simulink model "exemple_thermo_1"  (Simulink 8.1)
settings: Solver=ode4  StartTime=0.0  StopTime=10.0  FixedStep=1e-4  RelTol=1e-3
values from neighbouring files (symbols this model uses):
  Cp = 1000    [init_modele_thermo.m]
  Cv = 713    [init_modele_thermo.m]
  P0 = 1e5    (= 100000)    [init_modele_thermo.m]
  P1 = 1.05e5    (= 105000)    [init_modele_thermo.m]
  Pinit = 1e5    (= 100000)    [init_modele_thermo.m]
  r = 286.68    [init_modele_thermo.m]
  S_amont = pi/4*(5e-3)^2    (= 1.96349540849e-05)    [init_modele_thermo.m]
  S_aval = pi/4*(5e-3)^2    (= 1.96349540849e-05)    [init_modele_thermo.m]
  T0 = 300    [init_modele_thermo.m]
  T1 = 373    [init_modele_thermo.m]
  Tinit = 300    [init_modele_thermo.m]
  V = 1e-3    (= 0.001)    [init_modele_thermo.m]
settings Model: Creator=U243624  LastModifiedBy=U243624
settings DataIOCC: SignalLoggingSaveFormat=Dataset
settings OptimizationCC: ExpressionDepthLimit=128
settings DebuggingCC: FcnCallInpInsideContextMsg=EnableAllAsError
settings GRTTargetCC: CombineOutputUpdateFcns=on  GRTInterface=off

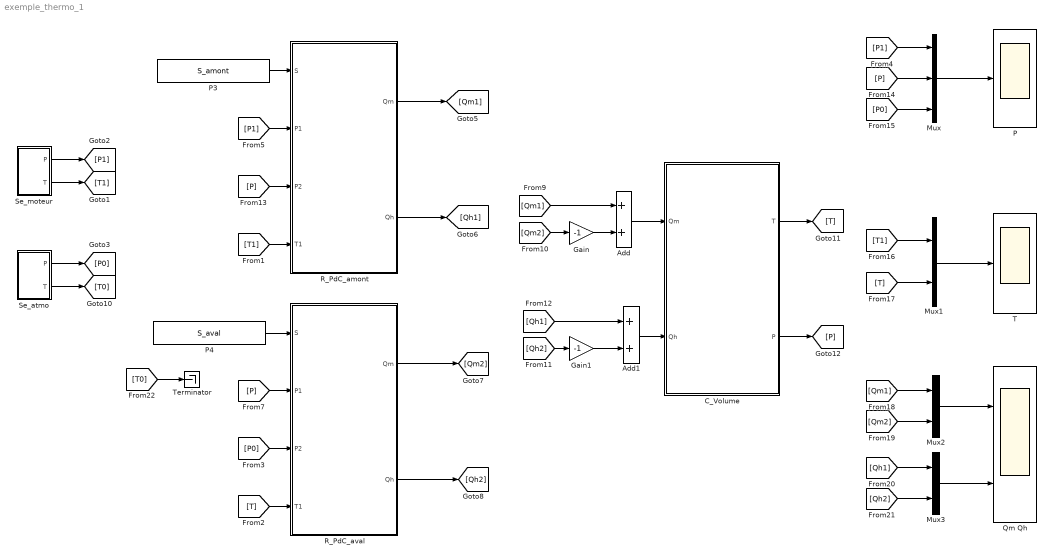
== system exemple_thermo_1 ==
  Add : Sum
  Add1 : Sum
  C_Volume : Subsystem
  Gain : Gain  Gain=-1
  Gain1 : Gain  Gain=-1
  Mux : Mux  Inputs=3
  Mux1 : Mux  Inputs=2
  Mux2 : Mux  Inputs=2
  Mux3 : Mux  Inputs=2
  "P " : Scope
  P3 : Constant  Value=S_amont
  P4 : Constant  Value=S_aval
  Qm Qh : Scope  NumInputPorts=2
      settings: YMin=-5~-5  YMax=5~5  SaveName=ScopeData2
  R_PdC_amont : Subsystem
  R_PdC_aval : Subsystem
  Se_atmo : Subsystem
  Se_moteur : Subsystem
  "T " : Scope
  Terminator : Terminator
  wires:
  Se_atmo/1(P) -> [P0]
  [P1] -> R_PdC_amont/2(P1)
  [P] -> R_PdC_amont/3(P2)
  [T1] -> R_PdC_amont/4(T1)
  R_PdC_amont/1(Qm) -> [Qm1]
  R_PdC_amont/2(Qh) -> [Qh1]
  P4/1 -> R_PdC_aval/1(S)
  [P] -> R_PdC_aval/2(P1)
  [P0] -> R_PdC_aval/3(P2)
  [T] -> R_PdC_aval/4(T1)
  R_PdC_aval/1(Qm) -> [Qm2]
  R_PdC_aval/2(Qh) -> [Qh2]
  [Qm1] -> Add/1
  [Qm2] -> Gain/1
  [Qh1] -> Add1/1
  [Qh2] -> Gain1/1
  Add/1 -> C_Volume/1(Qm)
  Add1/1 -> C_Volume/2(Qh)
  C_Volume/1(T) -> [T]
  C_Volume/2(P) -> [P]
  Gain/1 -> Add/2
  Gain1/1 -> Add1/2
  [P1] -> Mux/1
  [P] -> Mux/2
  [P0] -> Mux/3
  [T1] -> Mux1/1
  [T] -> Mux1/2
  Mux2/1 -> Qm Qh/1
  Mux/1 -> "P "/1
  Mux1/1 -> "T "/1
  [Qm1] -> Mux2/1
  [Qm2] -> Mux2/2
  Mux3/1 -> Qm Qh/2
  [Qh1] -> Mux3/1
  [Qh2] -> Mux3/2
  Se_moteur/1(P) -> [P1]
  Se_moteur/2(T) -> [T1]
  [T0] -> Terminator/1
  Se_atmo/2(T) -> [T0]
  P3/1 -> R_PdC_amont/1(S)

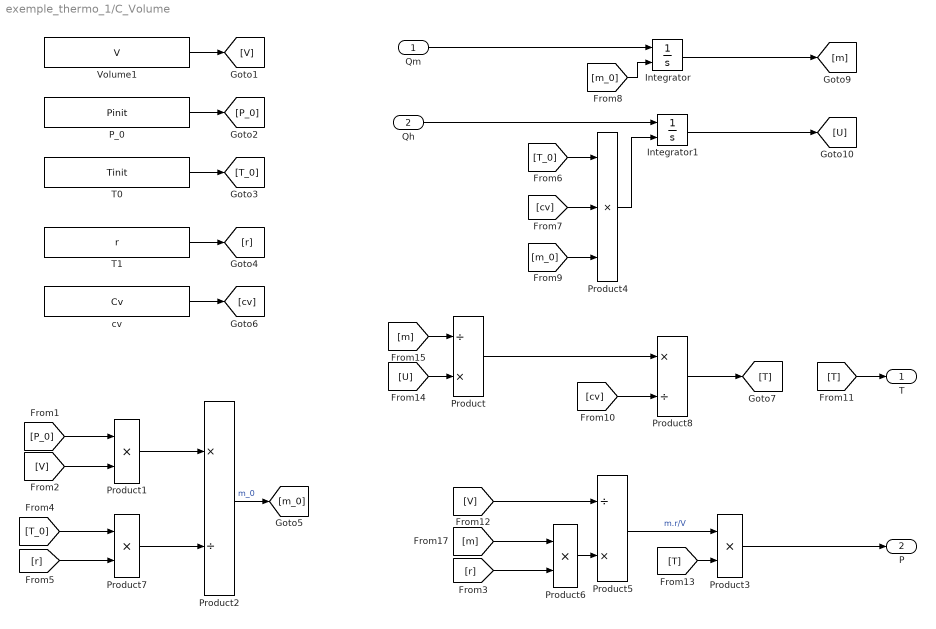
== system exemple_thermo_1/C_Volume ==
  Qm : Inport
  Qh : Inport  Port=2
  Integrator : Integrator  InitialConditionSource=external
  Integrator1 : Integrator  InitialConditionSource=external
  P_0 : Constant  Value=Pinit
  Product : Product  Inputs=/*  SaturateOnIntegerOverflow=on  RndMeth=Zero  InputSameDT=on  OutDataTypeStr=Inherit: Same as first input
  Product{1,3,6..7} (4 alike) : Product  SaturateOnIntegerOverflow=on  RndMeth=Zero  InputSameDT=on  OutDataTypeStr=Inherit: Same as first input
  Product2 : Product  Inputs=*/  SaturateOnIntegerOverflow=on  RndMeth=Zero  InputSameDT=on  OutDataTypeStr=Inherit: Same as first input
  Product4 : Product  Inputs=3  SaturateOnIntegerOverflow=on  RndMeth=Zero  InputSameDT=on  OutDataTypeStr=Inherit: Same as first input
  Product5 : Product  Inputs=/*  SaturateOnIntegerOverflow=on  RndMeth=Zero  InputSameDT=on  OutDataTypeStr=Inherit: Same as first input
  Product8 : Product  Inputs=*/  SaturateOnIntegerOverflow=on  RndMeth=Zero  InputSameDT=on  OutDataTypeStr=Inherit: Same as first input
  T0 : Constant  Value=Tinit
  T1 : Constant  Value=r
  Volume1 : Constant  Value=V
  cv : Constant  Value=Cv
  T : Outport
  P : Outport  Port=2
  wires:
  [V] -> Product5/1
  [T] -> T/1
  [cv] -> Product8/2
  Product4/1 -> Integrator1/2
  [m_0] -> Product4/3
  cv/1 -> [cv]
  [m_0] -> Integrator/2
  [cv] -> Product4/2
  [T_0] -> Product4/1
  Product2/1 -> [m_0]  "m_0"
  [r] -> Product7/2
  [T_0] -> Product7/1
  [r] -> Product6/2
  T1/1 -> [r]
  Product7/1 -> Product2/2
  Product1/1 -> Product2/1
  [V] -> Product1/2
  P_0/1 -> [P_0]
  T0/1 -> [T_0]
  [P_0] -> Product1/1
  Volume1/1 -> [V]
  Product3/1 -> P/1
  [T] -> Product3/2
  Product6/1 -> Product5/2
  Product5/1 -> Product3/1  "m.r/V"
  [m] -> Product6/1
  Integrator/1 -> [m]
  Qm/1 -> Integrator/1
  Qh/1 -> Integrator1/1
  Product8/1 -> [T]
  [U] -> Product/2
  Integrator1/1 -> [U]
  Product/1 -> Product8/1
  [m] -> Product/1

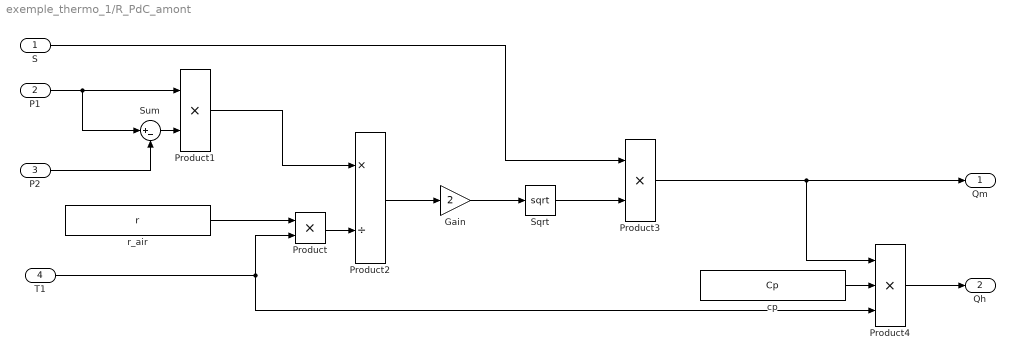
== system exemple_thermo_1/R_PdC_amont ==
  S : Inport
  P1 : Inport  Port=2
  P2 : Inport  Port=3
  T1 : Inport  Port=4
  Gain : Gain  Gain=2
  Product : Product
  Product1 : Product
  Product2 : Product  Inputs=*/
  Product3 : Product
  Product4 : Product  Inputs=3
  Sqrt : Sqrt  SaturateOnIntegerOverflow=on
  Sum : Sum  Inputs=|+-
  cp : Constant  Value=Cp
  r_air : Constant  Value=r
  Qm : Outport
  Qh : Outport  Port=2
  wires:
  P2/1 -> Sum/2
  Product1/1 -> Product2/1
  Product2/1 -> Gain/1
  Gain/1 -> Sqrt/1
  Product3/1 -> Product4/1, Qm/1
  r_air/1 -> Product/1
  P1/1 -> Sum/1, Product1/1
  Sqrt/1 -> Product3/2
  Sum/1 -> Product1/2
  S/1 -> Product3/1
  Product/1 -> Product2/2
  T1/1 -> Product4/3, Product/2
  cp/1 -> Product4/2
  Product4/1 -> Qh/1

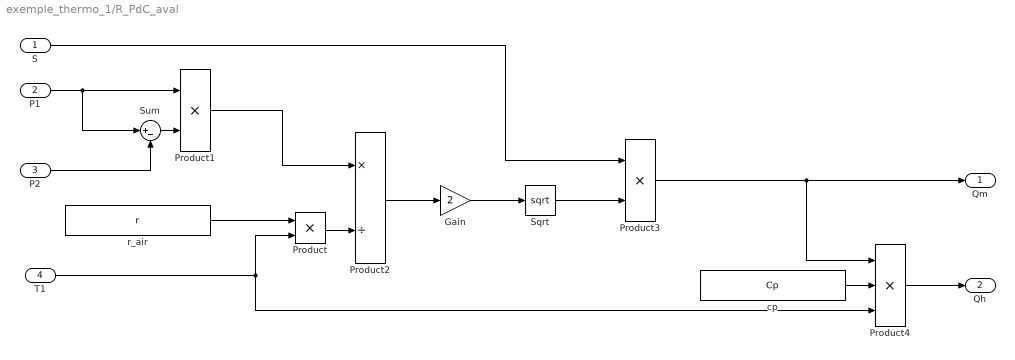
== system exemple_thermo_1/R_PdC_aval ==
  S : Inport
  P1 : Inport  Port=2
  P2 : Inport  Port=3
  T1 : Inport  Port=4
  Gain : Gain  Gain=2
  Product : Product
  Product1 : Product
  Product2 : Product  Inputs=*/
  Product3 : Product
  Product4 : Product  Inputs=3
  Sqrt : Sqrt  SaturateOnIntegerOverflow=on
  Sum : Sum  Inputs=|+-
  cp : Constant  Value=Cp
  r_air : Constant  Value=r
  Qm : Outport
  Qh : Outport  Port=2
  wires:
  Product4/1 -> Qh/1
  cp/1 -> Product4/2
  T1/1 -> Product/2, Product4/3
  Product/1 -> Product2/2
  S/1 -> Product3/1
  Sum/1 -> Product1/2
  Sqrt/1 -> Product3/2
  P1/1 -> Product1/1, Sum/1
  r_air/1 -> Product/1
  Product3/1 -> Qm/1, Product4/1
  Gain/1 -> Sqrt/1
  Product2/1 -> Gain/1
  Product1/1 -> Product2/1
  P2/1 -> Sum/2

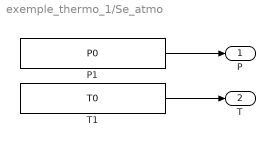
== system exemple_thermo_1/Se_atmo ==
  P1 : Constant  Value=P0
  T1 : Constant  Value=T0
  P : Outport
  T : Outport  Port=2
  wires:
  P1/1 -> P/1
  T1/1 -> T/1

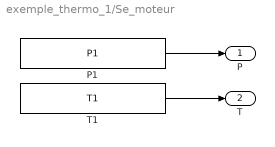
== system exemple_thermo_1/Se_moteur ==
  P1 : Constant  Value=P1
  T1 : Constant  Value=T1
  P : Outport
  T : Outport  Port=2
  wires:
  T1/1 -> T/1
  P1/1 -> P/1
